simulink library "Lib_PFSys_GenericACMotor_TMATS"  (R2018a)
settings: Solver=ode45  StartTime=0.0  StopTime=10.0  RelTol=1e-3  EnableMultiTasking=on
libraries: Lib_PF_ImpedanceAC_TMATS x1, Lib_PF_BusLoadDC_TMATS x1
Description:
  | Thomas Modules
settings Model: Creator=jwchapm2  LastModifiedBy=mebell
settings DataIOCC: LimitDataPoints=on  SaveFormat=Array
settings OptimizationCC: ExpressionDepthLimit=2147483647  LifeSpan=inf
settings DebuggingCC: UnderspecifiedInitializationDetection=Classic  MergeDetectMultiDrivingBlocksExec=none  SolverPrmCheckMsg=warning  StateNameClashWarn=warning  SFUnexpectedBacktrackingDiag=warning  SFNoUnconditionalDefaultTransitionDiag=warning  SFExecutionAtInitializationDiag=none
settings HardwareCC: ProdBitPerPointer=32  ProdBitPerSizeT=32  ProdBitPerPtrDiffT=32  ProdLargestAtomicFloat=None  ProdIntDivRoundTo=Undefined  ProdEndianess=Unspecified  ProdWordSize=32  ProdHWDeviceType=32-bit Generic
settings ModelReferenceCC: PropagateSignalLabelsOutOfModel=off
settings CodeAppCC: StateflowObjectComments=on
settings GRTTargetCC: TargetLangStandard=C89/C90 (ANSI)  GeneratePreprocessorConditionals=Disable all
settings ConfigComp: CovMetricSettings=dw  CovHtmlReporting=on  CovSaveCumulativeToWorkspaceVar=on  CovSaveSingleToWorkspaceVar=on  CovExternalEMLEnable=off

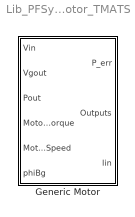
== system Lib_PFSys_GenericACMotor_TMATS ==
  Generic Motor : Subsystem  mask(Motor){X_C_TorqueVec_M=[0 1000 10000], Y_C_SpeedVec_M=[0 500 5000], T_C_EffArray_M=[0.5 0.5 0.5; 0.5 1 1; 0.5 1 1], R_M=0.01, L_M=0}
      mask prompts: X_C_TorqueVec_M "X_C_TorqueVec_M - Efficiency Table Torque Vector (X-axis)(nx1)"; Y_C_SpeedVec_M "Y_C_SpeedVec_M - Efficiency Table Speed Vector (Y-axis)(mx1)"; T_C_EffArray_M "T_C_EffArray_M - Efficiency Table Values (Eff = f(i, V)(nxm)"; R_M "R_M - Resistance"; L_M "L_M - Inductance"
      mask help: This block represents a generic motor with a standard resistive impedance of 0.01 Ohms and an efficiency table input.

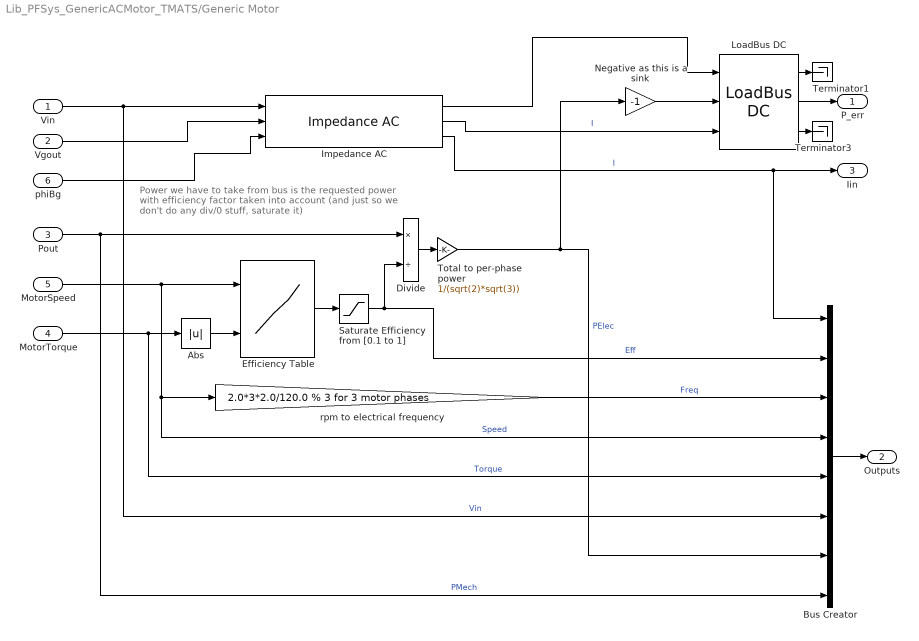
== system Lib_PFSys_GenericACMotor_TMATS/Generic Motor ==
  note: Power we have to take from bus is the requested power
      | with efficiency factor taken into account
      | (and just so we don't do any div/0 stuff, saturate it)
  Vin : Inport
  Vgout : Inport  Port=2
  Pout : Inport  Port=3
  MotorTorque : Inport  Port=4
  MotorSpeed : Inport  Port=5
  phiBg : Inport  Port=6
  Abs : Abs
  Bus Creator : BusCreator  Inputs=8
  Divide : Product  Inputs=*/
  Efficiency Table : Lookup_n-D  BreakpointsForDimension1=X_C_TorqueVec_M  BreakpointsForDimension2=Y_C_SpeedVec_M  Table=T_C_EffArray_M  ExtrapMethod=Clip  InternalRulePriority=Speed  RndMeth=Simplest  InputSameDT=on
  Impedance AC : Lib_PF_ImpedanceAC_TMATS/Impedance AC  R_M=100  X_M=0.015
  LoadBus DC : Lib_PF_BusLoadDC_TMATS/LoadBus DC  PeInEN_M=on  P_M=-2  BlkNm_M=double(gcb)
  Negative as this is a sink : Gain  Gain=-1
  Saturate Efficiency from [0.1 to 1] : Saturate  UpperLimit=1  LowerLimit=0.1
  Terminator1 : Terminator
  Terminator3 : Terminator
  Total to per-phase power : Gain  Gain=1/(sqrt(2)*sqrt(3))
  rpm to electrical frequency : Gain  Gain=2.0*3*2.0/120.0 % 3 for 3 motor phases
  P_err : Outport
  Outputs : Outport  Port=2
  Iin : Outport  Port=3
  wires:
  phiBg/1 -> Impedance AC/3
  Total to per-phase power/1 -> Bus Creator/7, Negative as this is a sink/1  "PElec"
  Negative as this is a sink/1 -> LoadBus DC/2
  Impedance AC/2 -> LoadBus DC/3  "I"
  Impedance AC/3 -> Bus Creator/1, Iin/1  "I"
  Impedance AC/1 -> LoadBus DC/1
  Vgout/1 -> Impedance AC/2
  Abs/1 -> Efficiency Table/2
  Bus Creator/1 -> Outputs/1
  rpm to electrical frequency/1 -> Bus Creator/3  "Freq"
  Divide/1 -> Total to per-phase power/1
  Saturate Efficiency from [0.1 to 1]/1 -> Divide/2, Bus Creator/2  "Eff"
  Efficiency Table/1 -> Saturate Efficiency from [0.1 to 1]/1
  MotorTorque/1 -> Bus Creator/5, Abs/1  "Torque"
  MotorSpeed/1 -> rpm to electrical frequency/1, Bus Creator/4, Efficiency Table/1  "Speed"
  LoadBus DC/3 -> Terminator3/1
  Vin/1 -> Bus Creator/6, Impedance AC/1  "Vin"
  Pout/1 -> Divide/1, Bus Creator/8  "PMech"
  LoadBus DC/2 -> P_err/1
  LoadBus DC/1 -> Terminator1/1
